simulink model "ex1impefk"  (R2025b)
settings: Solver=ode4  StartTime=0.0  StopTime=60  FixedStep=0.05  RelTol=1e-3
settings Model: Creator=Esteban  LastModifiedBy=Esteban

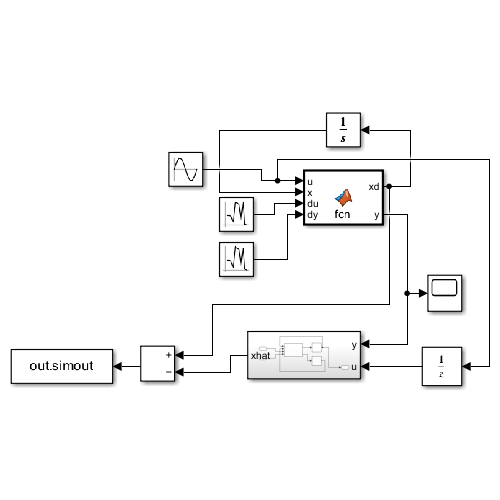
[thumbnail: Simulink's stored preview of the top-level diagram]
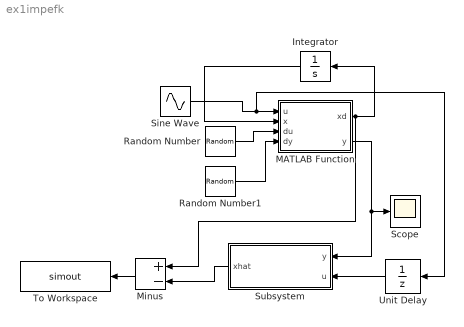
== system ex1impefk ==
  Integrator : Integrator  InitialCondition=[0;0]
  MATLAB Function : MATLAB Function  TreatAsAtomicUnit=on
  Minus : Sum  Inputs=+-
  Random Number : RandomNumber  Variance=0.01  SampleTime=0.05
  Random Number1 : RandomNumber  Variance=0.01  SampleTime=0.05
  Scope : Scope
  Sine Wave : Sin  Amplitude=1.1  Frequency=1.5  SampleTime=0
  Subsystem : Subsystem
  To Workspace : ToWorkspace  VariableName=simout  SaveFormat=Timeseries  SampleTime=-1
  Unit Delay : UnitDelay  SampleTime=-1  HasFrameUpgradeWarning=on
  wires:
  Random Number/1 -> MATLAB Function/3(du)
  Random Number1/1 -> MATLAB Function/4(dy)
  MATLAB Function/1(xd) -> Minus/1, Integrator/1
  Integrator/1 -> MATLAB Function/2(x)
  Sine Wave/1 -> Unit Delay/1, MATLAB Function/1(u)
  MATLAB Function/2(y) -> Scope/1, Subsystem/1(y)
  Unit Delay/1 -> Subsystem/2(u)
  Subsystem/1(xhat) -> Minus/2
  Minus/1 -> To Workspace/1

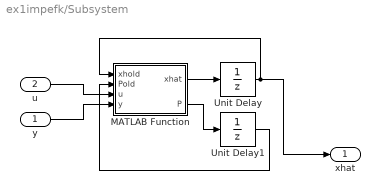
== system ex1impefk/Subsystem ==
  y : Inport
  u : Inport  Port=2
  MATLAB Function : MATLAB Function  TreatAsAtomicUnit=on
  Unit Delay : UnitDelay  InitialCondition=[0;0]  SampleTime=-1  HasFrameUpgradeWarning=on
  Unit Delay1 : UnitDelay  InitialCondition=zeros(2)  SampleTime=-1  HasFrameUpgradeWarning=on
  xhat : Outport
  wires:
  MATLAB Function/1(xhat) -> Unit Delay/1
  y/1 -> MATLAB Function/4(y)
  u/1 -> MATLAB Function/3(u)
  Unit Delay/1 -> MATLAB Function/1(xhold), xhat/1
  MATLAB Function/2(P) -> Unit Delay1/1
  Unit Delay1/1 -> MATLAB Function/2(Pold)

== matlab function ex1impefk/Subsystem/MATLAB Function ==
  data: xhold input; Pold input; u input; xhat output; y input; P output
function [xhat,P] = fcn(xhold,Pold,u,y)

tau = 0.1;

Qd=10*eye(2);
Rd=2;

f = [xhold(2)
     -6/5 * xhold(1)^3 + xhold(1) - u - 3*xhold(2) ];

J = [0 1
    -18/5*xhold(1)^2+1 -3];

F = eye(2) * tau*J;

%%

xp = xhold + tau*f;
Pp = F*Pold*F' + Qd;


H = [1 0];

S = H*Pp*H' + Rd;
K = Pp*H' /(S);

agg = y - H*xp;

xhat = xp + K*agg;
P = (eye(2)-K*H)*Pp;

== matlab function ex1impefk/MATLAB Function ==
  data: xd output; u input; y output; x input; du input; dy input
function [xd,y] = fcn(u,x,du,dy)

xd = [x(2)
     -6/5*x(1)^3+x(1)-u-3*x(2)+du];

y = x(1) + dy;
